simulink model "Problem_14"  (R2023a)
settings: Solver=VariableStepAuto  StartTime=0.0  StopTime=t  RelTol=1e-3
values from neighbouring files (symbols this model uses):
  alpha = 0    [Problem_14_script.m]
  Gamma_1 = diag([7 8 10])    [Problem_14_script.m]
  Gamma_2 = diag([1 1 1])    [Problem_14_script.m]
  k0 = param(1)    [Problem_14_script.m]
  k1 = param(4)    [Problem_14_script.m]
  lambda_0 = 100    [Problem_14_script.m]
  lambda_1 = 20    [Problem_14_script.m]
  theta_1_0 = [200 9 350]'    [Problem_14_script.m]
  theta_1_real = [k0*w0^2 2*xi0*w0 w0^2]    [Problem_14_script.m]
  theta_2_0 = [10 8 200]'    [Problem_14_script.m]
  w0 = param(2)    [Problem_14_script.m]
  w1 = param(5)    [Problem_14_script.m]
  xi0 = param(3)    [Problem_14_script.m]
  xi1 = param(6)    [Problem_14_script.m]
undefined symbols (not defined in the file or in its folder): k_0, k_1, w_0, w_1, xi_0, xi_1
settings Model: Creator=eliasoa  LastModifiedBy=eliasoa

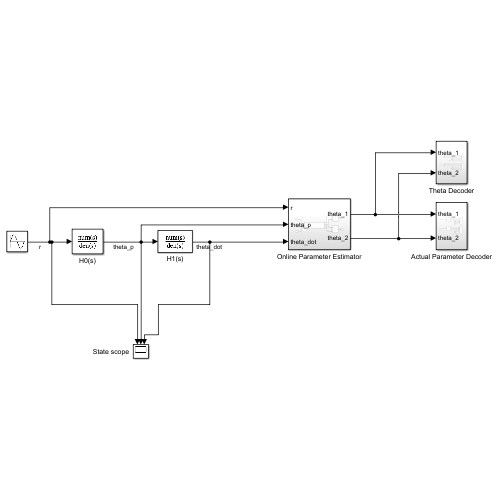
[thumbnail: Simulink's stored preview of the top-level diagram]
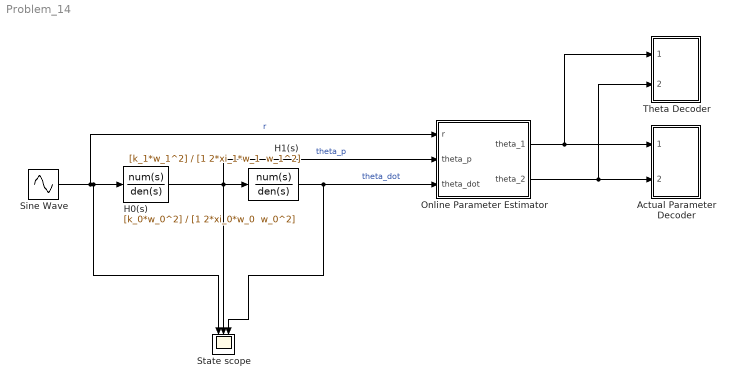
== system Problem_14 ==
  Actual Parameter Decoder : Subsystem
  H0(s) : TransferFcn  Numerator=[k_0*w_0^2]  Denominator="[1 2*xi_0*w_0  w_0^2]"
  H1(s) : TransferFcn  Numerator=[k_1*w_1^2]  Denominator="[1 2*xi_1*w_1  w_1^2]"
  Online Parameter Estimator : Subsystem
  Sine Wave : Sin  Amplitude=10  Bias=8  Frequency=0.2  SampleTime=0
  State scope : Scope  NumInputPorts=3
  Theta Decoder : Subsystem
  wires:
  H0(s)/1 -> State scope/2, H1(s)/1, Online Parameter Estimator/2(theta_p)  "theta_p"
  Sine Wave/1 -> State scope/1, H0(s)/1, Online Parameter Estimator/1(r)  "r"
  H1(s)/1 -> Online Parameter Estimator/3(theta_dot), State scope/3  "theta_dot"
  Online Parameter Estimator/1(theta_1) -> Theta Decoder/1(theta_1), Actual Parameter Decoder/1(theta_1)
  Online Parameter Estimator/2(theta_2) -> Theta Decoder/2(theta_2), Actual Parameter Decoder/2(theta_2)

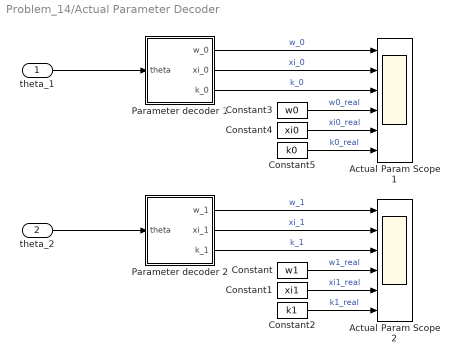
== system Problem_14/Actual Parameter Decoder ==
  theta_1 : Inport
  theta_2 : Inport  Port=2
  Actual Param Scope 1 : Scope  NumInputPorts=6
  Actual Param Scope 2 : Scope  NumInputPorts=6
  Constant : Constant  Value=w1
  Constant1 : Constant  Value=xi1
  Constant2 : Constant  Value=k1
  Constant3 : Constant  Value=w0
  Constant4 : Constant  Value=xi0
  Constant5 : Constant  Value=k0
  Parameter decoder 1 : MATLAB Function  TreatAsAtomicUnit=on
  Parameter decoder 2 : MATLAB Function  TreatAsAtomicUnit=on
  wires:
  Constant2/1 -> Actual Param Scope 2/6  "k1_real"
  Parameter decoder 2/1(w_1) -> Actual Param Scope 2/1  "w_1"
  Constant3/1 -> Actual Param Scope 1/4  "w0_real"
  Constant/1 -> Actual Param Scope 2/4  "w1_real"
  Constant1/1 -> Actual Param Scope 2/5  "xi1_real"
  Parameter decoder 1/2(xi_0) -> Actual Param Scope 1/2  "xi_0"
  Constant4/1 -> Actual Param Scope 1/5  "xi0_real"
  Parameter decoder 2/2(xi_1) -> Actual Param Scope 2/2  "xi_1"
  Parameter decoder 2/3(k_1) -> Actual Param Scope 2/3  "k_1"
  Constant5/1 -> Actual Param Scope 1/6  "k0_real"
  Parameter decoder 1/3(k_0) -> Actual Param Scope 1/3  "k_0"
  Parameter decoder 1/1(w_0) -> Actual Param Scope 1/1  "w_0"
  theta_1/1 -> Parameter decoder 1/1(theta)
  theta_2/1 -> Parameter decoder 2/1(theta)

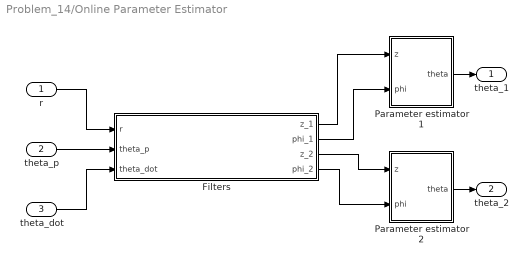
== system Problem_14/Online Parameter Estimator ==
  r : Inport
  theta_p : Inport  Port=2
  theta_dot : Inport  Port=3
  Filters : Subsystem
  Parameter estimator 1 : Subsystem
  Parameter estimator 2 : Subsystem
  theta_1 : Outport
  theta_2 : Outport  Port=2
  wires:
  Parameter estimator 1/1(theta) -> theta_1/1
  Filters/4(phi_2) -> Parameter estimator 2/2(phi)
  Filters/1(z_1) -> Parameter estimator 1/1(z)
  Filters/3(z_2) -> Parameter estimator 2/1(z)
  Filters/2(phi_1) -> Parameter estimator 1/2(phi)
  Parameter estimator 2/1(theta) -> theta_2/1
  r/1 -> Filters/1(r)
  theta_p/1 -> Filters/2(theta_p)
  theta_dot/1 -> Filters/3(theta_dot)

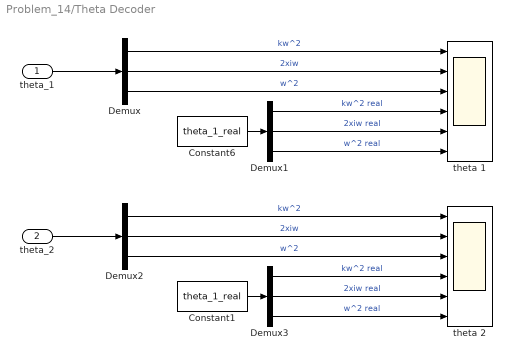
== system Problem_14/Theta Decoder ==
  theta_1 : Inport
  theta_2 : Inport  Port=2
  Constant1 : Constant  Value=theta_1_real
  Constant6 : Constant  Value=theta_1_real
  Demux{,1..3} (4 alike) : Demux  Outputs=3
  theta 1 : Scope  NumInputPorts=6
  theta 2 : Scope  NumInputPorts=6
  wires:
  Demux/2 -> theta 1/2  "2xiw"
  Constant1/1 -> Demux3/1
  Demux1/3 -> theta 1/6  "w^2 real"
  Demux1/1 -> theta 1/4  "kw^2 real"
  Demux/3 -> theta 1/3  "w^2"
  Demux1/2 -> theta 1/5  "2xiw real"
  Constant6/1 -> Demux1/1
  theta_1/1 -> Demux/1
  Demux3/2 -> theta 2/5  "2xiw real"
  Demux3/1 -> theta 2/4  "kw^2 real"
  Demux2/1 -> theta 2/1  "kw^2"
  Demux3/3 -> theta 2/6  "w^2 real"
  Demux2/3 -> theta 2/3  "w^2"
  Demux2/2 -> theta 2/2  "2xiw"
  Demux/1 -> theta 1/1  "kw^2"
  theta_2/1 -> Demux2/1

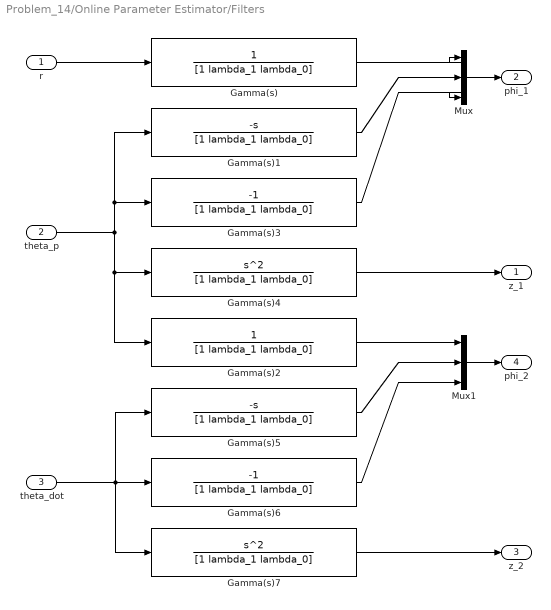
== system Problem_14/Online Parameter Estimator/Filters ==
  r : Inport
  theta_p : Inport  Port=2
  theta_dot : Inport  Port=3
  Gamma(s) : TransferFcn  Denominator=[1 lambda_1 lambda_0]
  Gamma(s)1 : TransferFcn  Numerator=[-1 0]  Denominator=[1 lambda_1 lambda_0]
  Gamma(s)2 : TransferFcn  Denominator=[1 lambda_1 lambda_0]
  Gamma(s)3 : TransferFcn  Numerator=[-1]  Denominator=[1 lambda_1 lambda_0]
  Gamma(s)4 : TransferFcn  Numerator=[1 0 0]  Denominator=[1 lambda_1 lambda_0]
  Gamma(s)5 : TransferFcn  Numerator=[-1 0]  Denominator=[1 lambda_1 lambda_0]
  Gamma(s)6 : TransferFcn  Numerator=[-1]  Denominator=[1 lambda_1 lambda_0]
  Gamma(s)7 : TransferFcn  Numerator=[1 0 0]  Denominator=[1 lambda_1 lambda_0]
  Mux : Mux  Inputs=3
  Mux1 : Mux  Inputs=3
  z_1 : Outport
  phi_1 : Outport  Port=2
  z_2 : Outport  Port=3
  phi_2 : Outport  Port=4
  wires:
  r/1 -> Gamma(s)/1
  theta_p/1 -> Gamma(s)4/1, Gamma(s)2/1, Gamma(s)3/1, Gamma(s)1/1
  Mux/1 -> phi_1/1
  Gamma(s)/1 -> Mux/1
  Gamma(s)1/1 -> Mux/2
  Gamma(s)3/1 -> Mux/3
  Gamma(s)2/1 -> Mux1/1
  Mux1/1 -> phi_2/1
  Gamma(s)4/1 -> z_1/1
  theta_dot/1 -> Gamma(s)5/1, Gamma(s)7/1, Gamma(s)6/1
  Gamma(s)5/1 -> Mux1/2
  Gamma(s)6/1 -> Mux1/3
  Gamma(s)7/1 -> z_2/1

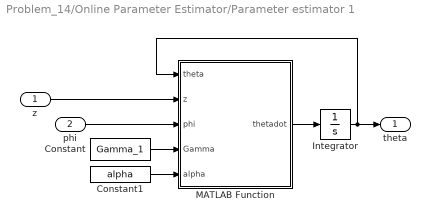
== system Problem_14/Online Parameter Estimator/Parameter estimator 1 ==
  z : Inport
  phi : Inport  Port=2
  Constant : Constant  Value=Gamma_1
  Constant1 : Constant  Value=alpha
  Integrator : Integrator  InitialCondition=theta_1_0
  MATLAB Function : MATLAB Function  TreatAsAtomicUnit=on
  theta : Outport
  wires:
  Constant1/1 -> MATLAB Function/5(alpha)
  Integrator/1 -> theta/1, MATLAB Function/1(theta)
  MATLAB Function/1(thetadot) -> Integrator/1
  Constant/1 -> MATLAB Function/4(Gamma)
  z/1 -> MATLAB Function/2(z)
  phi/1 -> MATLAB Function/3(phi)

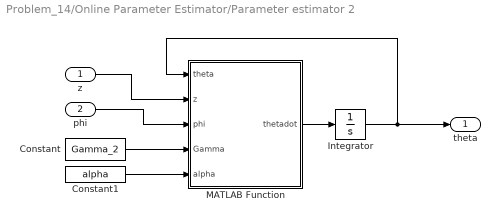
== system Problem_14/Online Parameter Estimator/Parameter estimator 2 ==
  z : Inport
  phi : Inport  Port=2
  Constant : Constant  Value=Gamma_2
  Constant1 : Constant  Value=alpha
  Integrator : Integrator  InitialCondition=theta_2_0
  MATLAB Function : MATLAB Function  TreatAsAtomicUnit=on
  theta : Outport
  wires:
  Constant1/1 -> MATLAB Function/5(alpha)
  Integrator/1 -> theta/1, MATLAB Function/1(theta)
  MATLAB Function/1(thetadot) -> Integrator/1
  Constant/1 -> MATLAB Function/4(Gamma)
  z/1 -> MATLAB Function/2(z)
  phi/1 -> MATLAB Function/3(phi)

== matlab function Problem_14/Online Parameter Estimator/Parameter estimator 1/MATLAB Function ==
  data: theta input; thetadot output; z input; phi input; Gamma input; alpha input
function thetadot = fcn(theta,z,phi,Gamma,alpha)
m2 = 1 + alpha*phi'*phi;
epsilon = (z-theta'*phi)/m2;
thetadot = Gamma * epsilon * phi;

== matlab function Problem_14/Online Parameter Estimator/Parameter estimator 2/MATLAB Function ==
  data: theta input; thetadot output; z input; phi input; Gamma input; alpha input
function thetadot = fcn(theta,z,phi,Gamma,alpha)
m2 = 1 + alpha*phi'*phi;
epsilon = (z-theta'*phi)/m2;
thetadot = Gamma * epsilon * phi;

== matlab function Problem_14/Actual Parameter Decoder/Parameter decoder 1 ==
  data: theta input; w_0 output; xi_0 output; k_0 output
function [w_0, xi_0, k_0] = fcn(theta)
theta_1 = theta(1); % kω^2
theta_2 = theta(2); % 2ξω
theta_3 = theta(3); % ω^2

w_0= sqrt(theta_3);
xi_0 = 1/(2*w_0)*theta_2;
k_0= theta_1/theta_3;

== matlab function Problem_14/Actual Parameter Decoder/Parameter decoder 2 ==
  data: theta input; w_1 output; xi_1 output; k_1 output
function [w_1, xi_1, k_1] = fcn(theta)
theta_1 = theta(1); % kω^2
theta_2 = theta(2); % 2ξω
theta_3 = theta(3); % ω^2

w_1= sqrt(theta_3);
xi_1 = 1/(2*w_1)*theta_2;
k_1= theta_1/theta_3;
